simulink model "floribot_task3"  (R2013a)
settings: Solver=FixedStepDiscrete  SolverMode=SingleTasking  StartTime=0.0  StopTime=inf  FixedStep=0.01  RelTol=1e-3
settings Model: Creator=Torsten  LastModifiedBy=Torsten
settings OptimizationCC: OptimizeModelRefInitCode=on  LifeSpan=Inf
settings RTWCC: SystemTargetFile=ert.tlc  GenCodeOnly=on  GenerateMakefile=off  TemplateMakefile=ert_default_tmf  Description=Embedded Coder  ProcessScript=ert_make_rtw_hook  TargetLang=C++
settings CodeAppCC: IgnoreCustomStorageClasses=off
settings ERTTargetCC: SupportNonFinite=off  SupportComplex=off  InlinedParameterPlacement=Hierarchical  ERTCustomFileTemplate=example_file_process.tlc

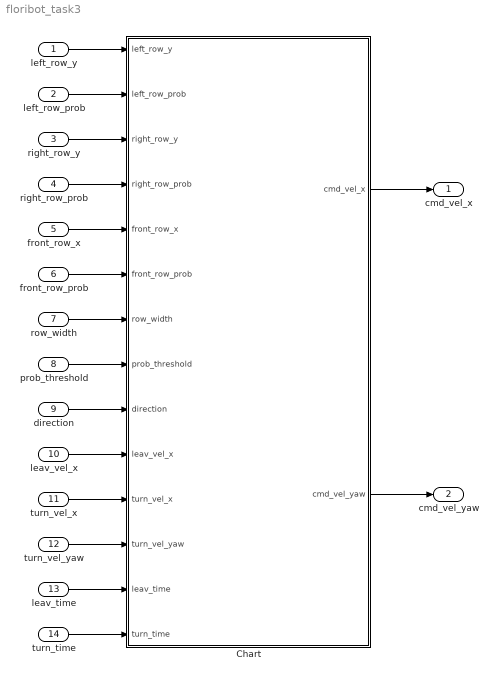
== system floribot_task3 ==
  left_row_y : Inport
  left_row_prob : Inport  Port=2
  right_row_y : Inport  Port=3
  right_row_prob : Inport  Port=4
  front_row_x : Inport  Port=5
  front_row_prob : Inport  Port=6
  row_width : Inport  Port=7
  prob_threshold : Inport  Port=8
  direction : Inport  Port=9
  leav_vel_x : Inport  Port=10
  turn_vel_x : Inport  Port=11
  turn_vel_yaw : Inport  Port=12
  leav_time : Inport  Port=13
  turn_time : Inport  Port=14
  Chart : Stateflow chart  TreatAsAtomicUnit=on
  cmd_vel_x : Outport
  cmd_vel_yaw : Outport  Port=2
  wires:
  Chart/1(cmd_vel_x) -> cmd_vel_x/1
  Chart/2(cmd_vel_yaw) -> cmd_vel_yaw/1
  left_row_y/1 -> Chart/1(left_row_y)
  left_row_prob/1 -> Chart/2(left_row_prob)
  right_row_y/1 -> Chart/3(right_row_y)
  right_row_prob/1 -> Chart/4(right_row_prob)
  front_row_x/1 -> Chart/5(front_row_x)
  front_row_prob/1 -> Chart/6(front_row_prob)
  row_width/1 -> Chart/7(row_width)
  prob_threshold/1 -> Chart/8(prob_threshold)
  direction/1 -> Chart/9(direction)
  leav_vel_x/1 -> Chart/10(leav_vel_x)
  turn_vel_x/1 -> Chart/11(turn_vel_x)
  turn_vel_yaw/1 -> Chart/12(turn_vel_yaw)
  leav_time/1 -> Chart/13(leav_time)
  turn_time/1 -> Chart/14(turn_time)

== stateflow chart floribot_task3/Chart ==
  state no_danger
    state inside_row
    state leaving_row
      during:
      cmd_vel_x = leav_vel_x;
      cmd_vel_yaw = 0;
    state turn_right
      during:
      cmd_vel_x = turn_vel_x;
      cmd_vel_yaw = -turn_vel_yaw;
    state turn_left
      during:
      cmd_vel_x = turn_vel_x;
      cmd_vel_yaw = turn_vel_yaw;
    (default) -> inside_row : /
        | count = 0;
    inside_row -> inside_row [order 8] : [left_row_prob<prob_threshold && right_row_prob<prob_threshold && front_row_prob<prob_threshold && count <= 10]/
        | count++;
        | cmd_vel_x =  0.2;
    inside_row -> inside_row [order 2] : [right_row_prob<prob_threshold && left_row_prob>prob_threshold &&  front_row_x > 0]/
        | cmd_vel_x = front_row_x/2;
        | cmd_vel_yaw = (left_row_y - row_width/2)*1.5;
    inside_row -> inside_row [order 1] : [right_row_prob<prob_threshold && left_row_prob>prob_threshold && front_row_x == 0]/
        | cmd_vel_x =  0.2;
        | cmd_vel_yaw = (left_row_y - row_width/2)*1.5;
    inside_row -> inside_row [order 7] : [right_row_prob>prob_threshold && left_row_prob<prob_threshold && front_row_x > 0]/
        | cmd_vel_x =  front_row_x/2;
        | cmd_vel_yaw = (right_row_y + row_width/2)*1.5;
    inside_row -> inside_row [order 5] : [right_row_prob>prob_threshold && left_row_prob<prob_threshold && front_row_x == 0]/
        | cmd_vel_x =  0.2;
        | cmd_vel_yaw = (right_row_y + row_width/2)*1.5;
    inside_row -> inside_row [order 6] : [left_row_prob>prob_threshold && right_row_prob>prob_threshold &&  front_row_x > 0]/
        | cmd_vel_x =  front_row_x/2;
        | cmd_vel_yaw = (left_row_y + right_row_y)/2*1.5;
    inside_row -> inside_row [order 3] : [left_row_prob>prob_threshold && right_row_prob>prob_threshold && front_row_x == 0]/
        | cmd_vel_x = 0.5;
        | cmd_vel_yaw = (left_row_y + right_row_y)/2*1.5;
    turn_right -> inside_row : [after(turn_time,sec) &&  right_row_y<0 &&  right_row_y>-row_width/2]/dir=-dir;
    turn_left -> inside_row : [after(turn_time,sec) && left_row_y>0 && left_row_y<row_width/2]/dir=-dir;
    inside_row -> leaving_row [order 4] : [left_row_prob<prob_threshold && right_row_prob<prob_threshold && front_row_prob<prob_threshold && count > 10]/count=0;
    leaving_row -> turn_left [order 2] : [after(leav_time,sec) && dir > 0]
    leaving_row -> turn_right [order 1] : [after(leav_time,sec) && dir < 0]
  state danger
    cmd_vel_x = 0;
    cmd_vel_yaw = 0;
  (default) -> no_danger : /dir = direction;
  no_danger -> danger : [front_row_x <= 0.2 && front_row_prob > prob_threshold]
  danger -> no_danger : [front_row_x > 0.2]
  data: left_row_y input double; left_row_prob input double; right_row_y input double; right_row_prob input double; front_row_x input double; front_row_prob input double; cmd_vel_x output double; cmd_vel_yaw output double; row_width input double; prob_threshold input double; direction input double; dir local double; leav_vel_x input double; turn_vel_x input double; turn_vel_yaw input double; count local int32; leav_time input double; turn_time input double
